simulink model "mux_init"  (R2021a)
settings: Solver=VariableStepAuto  StartTime=0.0  StopTime=10.0  RelTol=1e-3
settings Model: Creator=Aula  LastModifiedBy=Aula

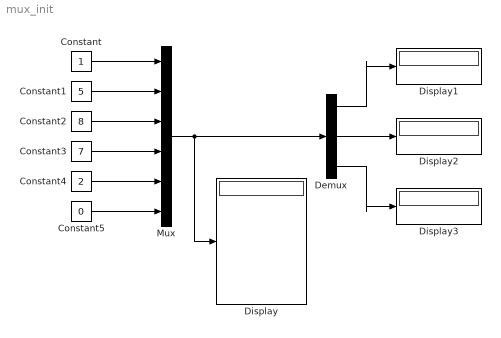
== system mux_init ==
  Constant : Constant
  Constant1 : Constant  Value=5
  Constant2 : Constant  Value=8
  Constant3 : Constant  Value=7
  Constant4 : Constant  Value=2
  Constant5 : Constant  Value=0
  Demux : Demux  Outputs=3
  Display{,1..3} (4 alike) : Display
  Mux : Mux  Inputs=6
  wires:
  Constant/1 -> Mux/1
  Constant1/1 -> Mux/2
  Constant2/1 -> Mux/3
  Constant3/1 -> Mux/4
  Constant4/1 -> Mux/5
  Constant5/1 -> Mux/6
  Mux/1 -> Display/1, Demux/1
  Demux/1 -> Display1/1
  Demux/2 -> Display2/1
  Demux/3 -> Display3/1
